simulink model "lab_2"  (R2020b)
settings: Solver=VariableStepAuto  StartTime=0.0  StopTime=10.0  RelTol=1e-3
InitFcn:
  | A = [0 1; 4 -6];
  | b = [3; 0];
  | Q = [1 0; 0 1];
  | k = 50;
  | Q = k * Q;
  | r = 100;
  | [K, P] = lqr(A, b, Q, r);
undefined symbols (not defined in the file): K
settings Model: Creator=Eugene  LastModifiedBy=Eugene

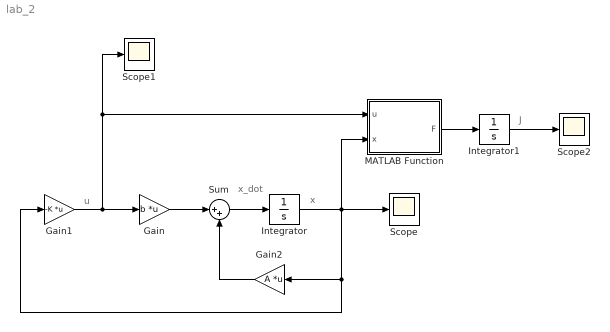
== system lab_2 ==
  note: J
  note: x
  note: x_dot
  note: u
  Gain : Gain  Gain=b  Multiplication=Matrix(K*u)
  Gain1 : Gain  Gain=-K  Multiplication=Matrix(K*u)
  Gain2 : Gain  Gain=A  Multiplication=Matrix(K*u)
  Integrator : Integrator  InitialCondition=[1; 0]
  Integrator1 : Integrator
  MATLAB Function : MATLAB Function  TreatAsAtomicUnit=on
  Scope : Scope
  Scope1 : Scope
  Scope2 : Scope
  Sum : Sum  Inputs=|++
  wires:
  Gain/1 -> Sum/1
  Sum/1 -> Integrator/1
  Integrator/1 -> Gain2/1, Gain1/1, MATLAB Function/2(x), Scope/1
  Gain2/1 -> Sum/2
  Gain1/1 -> Scope1/1, MATLAB Function/1(u), Gain/1
  MATLAB Function/1(F) -> Integrator1/1
  Integrator1/1 -> Scope2/1

== matlab function lab_2/MATLAB Function ==
  data: u input; F output; x input; Q parameter; r parameter
function F = fcn(u, x, Q, r)

F = x'*Q*x + r*u^2;
